simulink model "cartControl"  (R2017b)
settings: Solver=ode45  StartTime=0.0  StopTime=10.0  RelTol=1e-3  EnableMultiTasking=on
StopFcn:
  | if(exist('Q'))
  | 
  | pause_time = 0.001;
  | pause_on = 1;
  | 
  | figure(2)
  | h=uicontrol(gcf,'style','pushbutton','String','PLAY','position',[175 5 200 30]);
  | set(h,'callback','if(pause_on == 1); for i=1:size(Q.Data,1); plot(Rob, Q.Data(i,:));pause(pause_time); end; end; if(pause_on == 0); for i=1:size(Q.Data,1) plot(Rob, Q.Data(i,:)); end; end;');
  | 
  | h=uicontrol(gcf,'style','pushbutton','String','make slower','position',[50 5 100 30]);
  | set(h,'callback','pause_time = pause_time*2; if(pause_time>1e-4) pause_on = 1; end');
  | 
  | h=uicontrol(gcf,'style','pushbutton','String','make faster','position',[400 5 100 30]);
  | set(h,'callback','if(pause_time<1e-4) pause_on = 0; else; pause_time = pause_time/2; end ');
  | 
  | set(gcf, 'toolbar', 'figure')
  | 
  | end
model workspace (MAT data in the model file):
  Rob = SerialLink
  Rob.name = 'three link'
  Rob.gravity = [0; 0; 9.81]
  Rob.base = SE3
  Rob.base.data = [1  0  0  0; 0  1  0  0; 0  0  1  0; 0  0  0  1]
  Rob.tool = SE3
  Rob.tool.data = [1  0  0  0; 0  1  0  0; 0  0  1  0; 0  0  0  1]
  Rob.fast = 0
  Rob.n = 3
  Rob.links(1) = Link
  Rob.links(1).d = 0
  Rob.links(1).alpha = 0
  Rob.links(1).a = 4
  Rob.links(1).jointtype = 'R'
  Rob.links(1).mdh = 0
  Rob.links(1).offset = 0
  Rob.links(1).flip = 0
  Rob.links(1).m = 0
  Rob.links(1).r = [0 0 0]
  Rob.links(1).I = [0  0  0; 0  0  0; 0  0  0]
  Rob.links(1).Jm = 0
  Rob.links(1).B = 0
  Rob.links(1).Tc = [0 0]
  Rob.links(1).G = 0
  Rob.links(2) = Link
  Rob.links(2).d = 0
  Rob.links(2).alpha = 0
  Rob.links(2).a = 3
  Rob.links(2).jointtype = 'R'
  Rob.links(2).mdh = 0
  Rob.links(2).offset = 0
  Rob.links(2).flip = 0
  Rob.links(2).m = 0
  Rob.links(2).r = [0 0 0]
  Rob.links(2).I = [0  0  0; 0  0  0; 0  0  0]
  Rob.links(2).Jm = 0
  Rob.links(2).B = 0
  Rob.links(2).Tc = [0 0]
  Rob.links(2).G = 0
  Rob.links(3) = Link
  Rob.links(3).d = 0
  Rob.links(3).alpha = 0
  Rob.links(3).a = 2
  Rob.links(3).jointtype = 'R'
  Rob.links(3).mdh = 0
  Rob.links(3).offset = 0
  Rob.links(3).flip = 0
  Rob.links(3).m = 0
  Rob.links(3).r = [0 0 0]
  Rob.links(3).I = [0  0  0; 0  0  0; 0  0  0]
  Rob.links(3).Jm = 0
  Rob.links(3).B = 0
  Rob.links(3).Tc = [0 0]
  Rob.links(3).G = 0
  Rob.mdh = 0
undefined symbols (not defined in the file): fkine, jacob0, transl
settings Model: Creator=user  LastModifiedBy=c.chawla
settings DataIOCC: LimitDataPoints=on  SaveFormat=Array
settings OptimizationCC: LifeSpan=inf
settings DebuggingCC: UnderspecifiedInitializationDetection=Classic  MergeDetectMultiDrivingBlocksExec=none  SolverPrmCheckMsg=warning  SFUnexpectedBacktrackingDiag=warning  SFNoUnconditionalDefaultTransitionDiag=warning  SFExecutionAtInitializationDiag=none
settings HardwareCC: ProdBitPerPointer=32  ProdBitPerSizeT=32  ProdBitPerPtrDiffT=32  ProdLargestAtomicFloat=None  ProdIntDivRoundTo=Undefined  ProdEndianess=Unspecified  ProdWordSize=32  ProdHWDeviceType=32-bit Generic
settings ModelReferenceCC: PropagateSignalLabelsOutOfModel=off
settings CodeAppCC: StateflowObjectComments=on
settings GRTTargetCC: TargetLangStandard=C89/C90 (ANSI)  GeneratePreprocessorConditionals=Disable all
settings ConfigComp: CovMetricSettings=dw  CovHtmlReporting=on  CovSaveCumulativeToWorkspaceVar=on  CovSaveSingleToWorkspaceVar=on  CovExternalEMLEnable=off  CovSFcnEnable=off

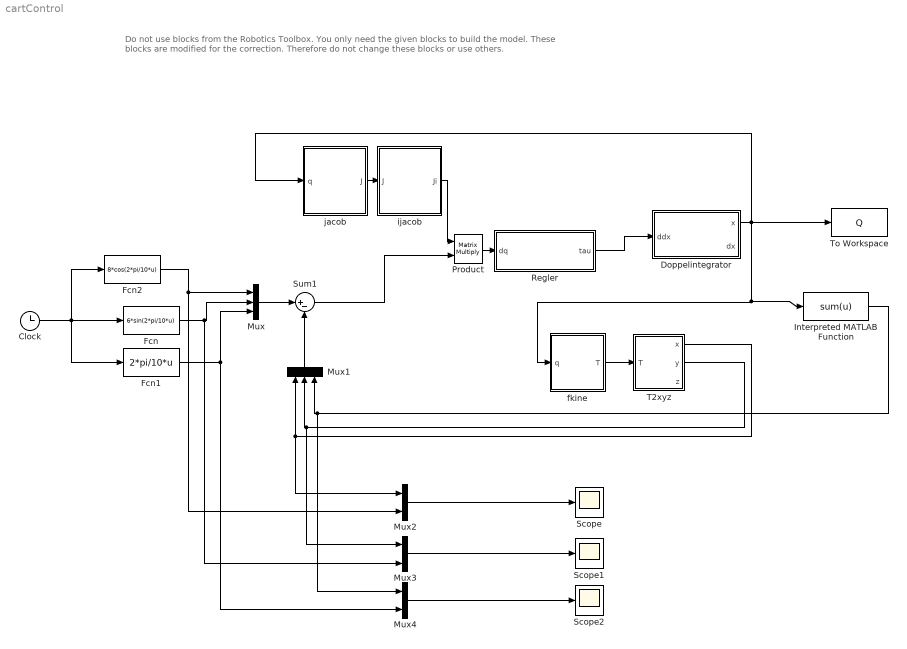
== system cartControl ==
  note: Do not use blocks from the Robotics Toolbox. You only need the given blocks to build the model.
      | These blocks are modified for the correction. Therefore do not change these blocks or use others.
  Clock : Clock
  Doppelintegrator : Subsystem  LoadFcn=set_param(gcb,'Name','Doppelintegrator');  InitFcn=set_param(gcb,'Name','Doppelintegrator');
      mask Display: dpoly([1],[1 0 0], 's')
  Fcn : Fcn  Expr=6*sin(2*pi/10*u)
  Fcn1 : Fcn  Expr=2*pi/10*u
  Fcn2 : Fcn  Expr=8*cos(2*pi/10*u)
  Interpreted MATLAB Function : MATLABFcn  MATLABFcn=sum(u)
  Mux : Mux  Inputs=3
  Mux1 : Mux  Inputs=3
  Mux2 : Mux  Inputs=2
  Mux3 : Mux  Inputs=2
  Mux4 : Mux  Inputs=2
  Product : Product  Multiplication=Matrix(*)
  Regler : Subsystem  LoadFcn=set_param(gcb,'Name','Regler');  InitFcn=set_param(gcb,'Name','Regler');
      mask Display: disp('PD-Regler')
  Scope : Scope
  Scope1 : Scope
  Scope2 : Scope
  Sum1 : Sum  Inputs=|+-
  T2xyz : Subsystem  LoadFcn=set_param(gcb,'Name','T2xyz');  InitFcn=set_param(gcb,'Name','T2xyz');
      mask help: Convert transform to xyz scalars
  To Workspace : ToWorkspace  VariableName=Q  SaveFormat=Timeseries  SampleTime=-1
  fkine : Subsystem  mask{robot=Rob}
      mask prompts: robot "SerialLink object"
      mask help: Robot forward kinematics.
  ijacob : Subsystem  LoadFcn=set_param(gcb,'Name','ijacob');  InitFcn=set_param(gcb,'Name','ijacob');
      mask help: Robot pseudoinverse Jacobian for world coordinates.
      mask Display:
      | text(0.4, 0.7, 'J', 'verticalAlignment', 'top', 'horizontalAlignment', 'left')
      | text(0.65, 0.65, '-1', 'verticalAlignment', 'bottom', 'horizontalAlignment', 'right')
      | port_label('input', 1, 'J');
      | port_label('output', 1, 'Ji')
  jacob : Subsystem  LoadFcn=set_param(gcb,'Name','jacob');  InitFcn=|  mask{robot=Rob}
      | set_param(gcb,'Name','jacob');
      | 
      | if(~any(strcmp(who,'Testumgebung')))
      | 
      | if(~strcmp(get_param(gcb,'Robot'),'Rob'))
      | set_param(gcb,'Robot','Rob');
      | warning('Verändern sie nichts in der Funktion jacob.')
      | end
      | 
      | end
      mask prompts: robot "SerialLink object"
      mask help: Robot Jacobian for end-effector coordinates
      mask init:
      | n=robot.n;
      mask Display:
      | text(0.4, 0.7, 'J', 'verticalAlignment', 'top', 'horizontalAlignment', 'left')
      | text(0.4, 0.7, '0', 'verticalAlignment', 'bottom', 'horizontalAlignment', 'right')
      | text(0.5, 0.2, robot.name,  'horizontalAlignment', 'center')
      | port_label('input', 1, 'q')
      | port_label('output', 1, 'J')
  wires:
  Clock/1 -> Fcn1/1, Fcn2/1, Fcn/1
  fkine/1(T) -> T2xyz/1(T)
  jacob/1(J) -> ijacob/1(J)
  Doppelintegrator/1(x) -> Interpreted MATLAB Function/1, fkine/1(q), jacob/1(q), To Workspace/1
  ijacob/1(Ji) -> Product/1
  Product/1 -> Regler/1(dq)
  Fcn2/1 -> Mux2/2, Mux/1
  Fcn/1 -> Mux3/2, Mux/2
  Fcn1/1 -> Mux4/2, Mux/3
  Mux/1 -> Sum1/1
  Mux1/1 -> Sum1/2
  Interpreted MATLAB Function/1 -> Mux4/1, Mux1/3
  T2xyz/1(x) -> Mux2/1, Mux1/1
  T2xyz/2(y) -> Mux3/1, Mux1/2
  Sum1/1 -> Product/2
  Mux3/1 -> Scope1/1
  Mux2/1 -> Scope/1
  Mux4/1 -> Scope2/1
  Regler/1(tau) -> Doppelintegrator/1(ddx)

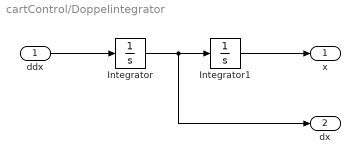
== system cartControl/Doppelintegrator ==
  ddx : Inport
  Integrator : Integrator  InitialCondition=[0 0 0]'
  Integrator1 : Integrator  InitialCondition=[-26.3845 62.7207 -36.3362]'/180*pi
  x : Outport
  dx : Outport  Port=2
  wires:
  Integrator/1 -> dx/1, Integrator1/1
  Integrator1/1 -> x/1
  ddx/1 -> Integrator/1

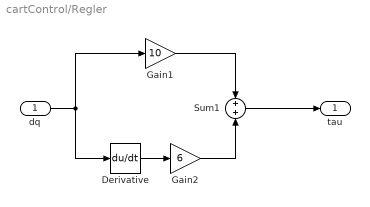
== system cartControl/Regler ==
  dq : Inport
  Derivative : Derivative
  Gain1 : Gain  Gain=10
  Gain2 : Gain  Gain=6
  Sum1 : Sum  Inputs=+|+
  tau : Outport
  wires:
  Sum1/1 -> tau/1
  Gain1/1 -> Sum1/1
  Gain2/1 -> Sum1/2
  dq/1 -> Derivative/1, Gain1/1
  Derivative/1 -> Gain2/1

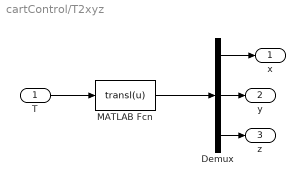
== system cartControl/T2xyz ==
  T : Inport
  Demux : Demux  Outputs=3
  MATLAB Fcn : MATLABFcn  MATLABFcn=transl(u)  OutputDimensions=3
  x : Outport
  y : Outport  Port=2
  z : Outport  Port=3
  wires:
  Demux/3 -> z/1
  Demux/2 -> y/1
  Demux/1 -> x/1
  MATLAB Fcn/1 -> Demux/1
  T/1 -> MATLAB Fcn/1

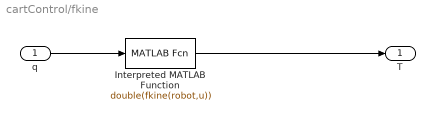
== system cartControl/fkine ==
  q : Inport
  Interpreted MATLAB Function : MATLABFcn  MATLABFcn=double(fkine(robot,u))  OutputDimensions=[4 4]  Output1D=off
  T : Outport
  wires:
  q/1 -> Interpreted MATLAB Function/1
  Interpreted MATLAB Function/1 -> T/1

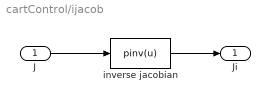
== system cartControl/ijacob ==
  J : Inport
  inverse jacobian : MATLABFcn  MATLABFcn=pinv(u)  Output1D=off
  Ji : Outport
  wires:
  J/1 -> inverse jacobian/1
  inverse jacobian/1 -> Ji/1

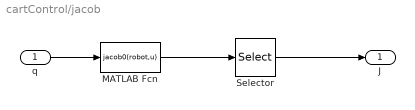
== system cartControl/jacob ==
  q : Inport
  MATLAB Fcn : MATLABFcn  MATLABFcn=jacob0(robot,u)  OutputDimensions=[6 n]  Output1D=off
  Selector : Selector  NumberOfDimensions=2  InputPortWidth=3  IndexOptions=Index vector (dialog),Index vector (dialog)  Indices=[1 2 6],[1 2 3]  OutputSizes=1,1
  J : Outport
  wires:
  q/1 -> MATLAB Fcn/1
  MATLAB Fcn/1 -> Selector/1
  Selector/1 -> J/1
